simulink model "Paper_Simulation"  (R2020a)
settings: Solver=VariableStepAuto  StartTime=0.0  StopTime=1  RelTol=1e-3
model workspace (MAT data in the model file):
  Wo = 1
  wfinal = Simulink.Parameter
  wfinal.DataType = 'auto'
  wfinal.Dimensions = [0 0]
undefined symbols (not defined in the file): fdesignblkfcn, gcbh, T1, T2, Tf
libraries: powerlib_meascontrol x3, simulink x2, eeSinusoidalMeasurementV2 x1
settings Model: Creator=Ayush Agrawal  LastModifiedBy=Ayush Agrawal
settings DebuggingCC: AlgebraicLoopMsg=none

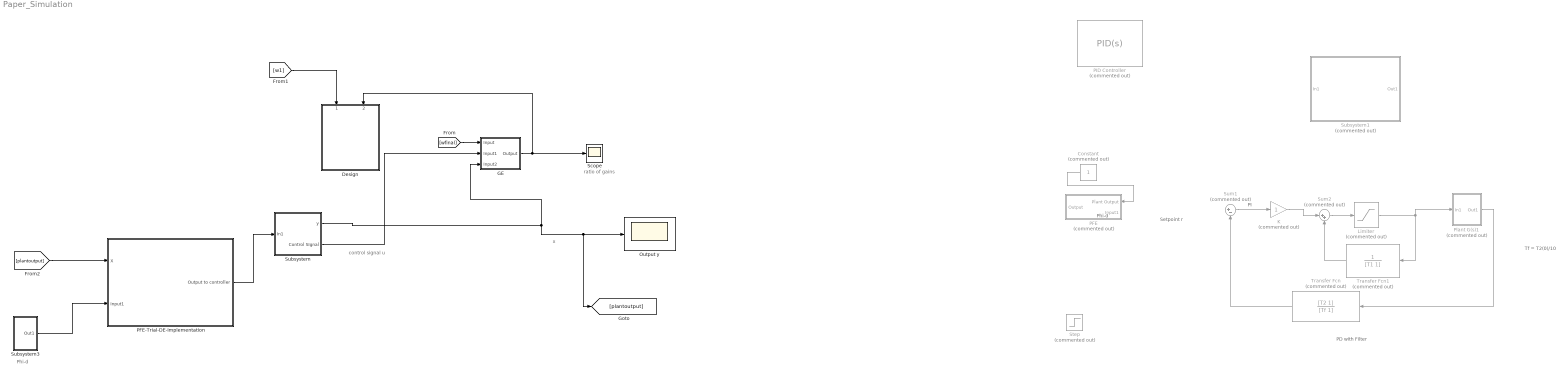
== system Paper_Simulation ==
  note: ratio of gains
  note: x
  note: Phi-d
  note: Phi-d
  note: control signal
      |         u
  note: Setpoint r
  note: PI
  note: PD with Filter
  note: Tf = T2(0)/10
  Constant : Constant  Commented=on
  Design : Subsystem  mask{a=1.5}
  GE : Subsystem  mask{winitial=10}
  K : Gain  Commented=on
  Limiter : Saturate  Commented=on
  Output y : Scope
  PFE : Subsystem  Commented=on
  PFE-Trial-DE-Implementation : Subsystem  mask{winitial=10}
  PID Controller : simulink/Continuous/PID Controller  Commented=on  Controller=PID  Form=Parallel  TimeDomain=Continuous-time  UseExternalTs=off  SampleTime=-1  IntegratorMethod=Forward Euler  FilterMethod=Forward Euler  ControllerParametersSource=internal  P=1  I=1  D=0  UseFilter=on  N=100  TunerSelectOption=Transfer Function Based (PID Tuner App)  InitialConditionSource=internal  InitialConditionForIntegrator=0  InitialConditionForFilter=0  DifferentiatorICPrevScaledInput=0  ExternalReset=none  TrackingMode=off  Kt=1  LimitOutput=off  UpperSaturationLimit=inf  LowerSaturationLimit=-inf  LinearizeAsGain=on  AntiWindupMode=none  Kb=1  POutMin=[]  POutMax=[]  IOutMin=[]  IOutMax=[]  DOutMin=[]  DOutMax=[]  NOutMin=[]  NOutMax=[]  SumOutMin=[]  SumOutMax=[]  SaturationOutMin=[]  SaturationOutMax=[]  PParamMin=[]  PParamMax=[]  IParamMin=[]  IParamMax=[]  DParamMin=[]  DParamMax=[]  NParamMin=[]  NParamMax=[]  KbParamMin=[]  KbParamMax=[]  KtParamMin=[]  KtParamMax=[]  KbOutMin=[]  KbOutMax=[]  KtOutMin=[]  KtOutMax=[]  IntegratorOutMin=[]  IntegratorOutMax=[]  FilterOutMin=[]  FilterOutMax=[]  SumI1OutMin=[]  SumI1OutMax=[]  SumI2OutMin=[]  SumI2OutMax=[]  SumI3OutMin=[]  SumI3OutMax=[]  SumI4OutMin=[]  SumI4OutMax=[]  SumDOutMin=[]  SumDOutMax=[]  DifferentiatorOutMin=[]  DifferentiatorOutMax=[]  FilterDiffOutCoefMin=[]  FilterDiffOutCoefMax=[]  ReciprocalOutMin=[]  ReciprocalOutMax=[]  SumDenOutMin=[]  SumDenOutMax=[]  SumNumOutMin=[]  SumNumOutMax=[]  DivideOutMin=[]  DivideOutMax=[]  UdiffTsProdOutMin=[]  UdiffTsProdOutMax=[]  NTsProdOutMin=[]  NTsProdOutMax=[]  UintegralTsProdOutMin=[]  UintegralTsProdOutMax=[]  UngainTsProdOutMin=[]  UngainTsProdOutMax=[]  IntegratorContinuousStateAttributes=''  IntegratorStateMustResolveToSignalObject=off  IntegratorRTWStateStorageClass=Auto  FilterContinuousStateAttributes=''  FilterStateMustResolveToSignalObject=off  FilterRTWStateStorageClass=Auto  ParallelPVariant=InternalParameters  IdealPVariant=Disabled  IVariant=InternalParameters  DVariant=InternalParameters  IntegratorVariant=Continuous  SatVariant=Disabled  AWVariant=Passthrough  PCopyVariant=Disabled  TRVariant=Disabled  FdbkBlocksVariant=Forward  IdealPFdbkVariant=Disabled  SatFdbkVariant=Disabled  DerivativeFilterVariant=ContFilter  NVariant=InternalParameters  NCopyVariant=Disabled  FilterICVariant=InternalICsFilter  IntegratorICVariant=InternalICs  ExternalResetVariant=Disabled  TRSumVariant=Passthrough  SumFdbkVariant=Disabled  SumVariant=Sum_PID  TsampFilterVariant=InternalTs  TsampNgainVariant=Passthrough  TsampIntegralVariant=Passthrough
  Plant G(s)1 : Subsystem  Commented=on
  Scope : Scope
  Step : Step  Commented=on  SampleTime=0
  Subsystem : Subsystem  mask{Ti=0, r=0.25}
  Subsystem1 : Subsystem  Commented=on
  Subsystem3 : Subsystem  mask{Phid=10}
      mask prompts: Phid "Phi-d"
  Sum1 : Sum  Commented=on  Inputs=|+-
  Sum2 : Sum  Commented=on  Inputs=|++
  Transfer Fcn : TransferFcn  Commented=on  Numerator=[T2 1]  Denominator=[Tf 1]
  Transfer Fcn1 : TransferFcn  Commented=on  Denominator=[T1 1]
  wires:
  Subsystem/1(y) -> GE/3(Input2), [plantoutput], Output y/1
  Sum2/1 -> Limiter/1
  Plant G(s)1/1(Out1) -> Transfer Fcn/1
  Limiter/1 -> Transfer Fcn1/1, Plant G(s)1/1(In1)
  Sum1/1 -> K/1
  Transfer Fcn/1 -> Sum1/2
  K/1 -> Sum2/1
  Transfer Fcn1/1 -> Sum2/2
  [wfinal] -> GE/1(Input)
  GE/1(Output) -> Scope/1, Design/2(Plant Gain Amplitude)
  [w1] -> Design/1(PFE O/P frequency)
  Constant/1 -> PFE/1(Plant Output)
  Subsystem3/1(Out1) -> PFE-Trial-DE-Implementation/2(Input1)
  [plantoutput] -> PFE-Trial-DE-Implementation/1(X)
  PFE-Trial-DE-Implementation/1(Output to controller) -> Subsystem/1(In1)
  Subsystem/2(Control SIgnal) -> GE/2(Input1)

== system Paper_Simulation/Design ==
  PFE O/P frequency : Inport
  Plant Gain Amplitude : Inport  Port=2
  Scope : Scope
  Scope1 : Scope
  Subsystem : Subsystem
  tag scope: K=global, Ti=global
  wires:
  PFE O/P frequency/1 -> Subsystem/1(PFE O/P freq)
  Plant Gain Amplitude/1 -> Subsystem/2(Input)
  Subsystem/1(K) -> Scope/1, [K]
  Subsystem/2(Ti) -> Scope1/1, [Ti]

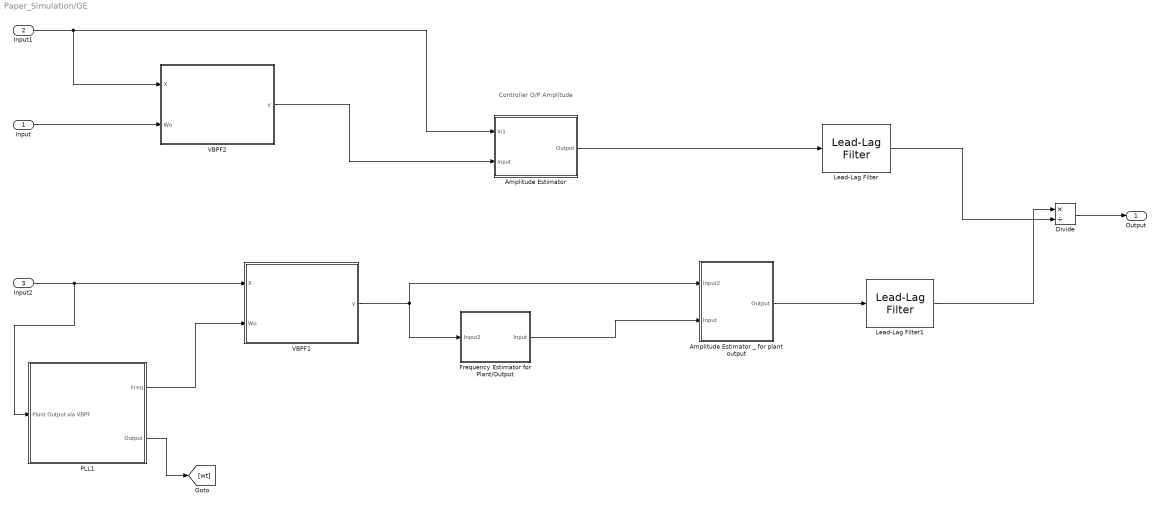
== system Paper_Simulation/GE ==
  note: Controller O/P Amplitude
  Input : Inport
  Input1 : Inport  Port=2
  Input2 : Inport  Port=3
  Amplitude Estimator : Subsystem
  Amplitude Estimator _ for plant output : Subsystem
  Divide : Product  Inputs=*/
  Frequency Estimator for Plant/Output : Subsystem
  Lead-Lag Filter : powerlib_meascontrol/Filters/Lead-Lag Filter  T1=0  T2=10/winitial  Vdc_Init=0  Ts=0
      settings: SourceProductBaseCode=PS
  Lead-Lag Filter1 : powerlib_meascontrol/Filters/Lead-Lag Filter  T1=0  T2=10/winitial  Vdc_Init=0  Ts=0
      settings: SourceProductBaseCode=PS
  PLL1 : Subsystem
  VBPF1 : Subsystem
  VBPF2 : Subsystem
  Output : Outport
  wires:
  Input1/1 -> VBPF2/1(X), Amplitude Estimator/1(In1)
  Input2/1 -> PLL1/1(Plant Output via VBPF), VBPF1/1(X)
  Amplitude Estimator/1(Output) -> Lead-Lag Filter/1
  Amplitude Estimator _ for plant output/1(Output) -> Lead-Lag Filter1/1
  Divide/1 -> Output/1
  Lead-Lag Filter1/1 -> Divide/1
  Lead-Lag Filter/1 -> Divide/2
  Frequency Estimator for Plant/Output/1(Input) -> Amplitude Estimator _ for plant output/2(Input)
  PLL1/1(Freq) -> VBPF1/2(Wo)
  PLL1/2(Output) -> [wt]
  Input/1 -> VBPF2/2(Wo)
  VBPF2/1(y) -> Amplitude Estimator/2(Input)
  VBPF1/1(y) -> Amplitude Estimator _ for plant output/1(Input2), Frequency Estimator for Plant/Output/1(Input2)

== system Paper_Simulation/PFE ==
  note: Phi-d
  Plant Output : Inport
  Input1 : Inport  Port=2
  PLL : Subsystem
  Subsystem : Subsystem  Commented=on
  Sum1 : Sum  Inputs=|+-
  VBPF1 : Subsystem
  Output : Outport
  wires:
  Plant Output/1 -> VBPF1/1(X)
  PLL/1(Output) -> Sum1/1
  Input1/1 -> Sum1/2
  Sum1/1 -> Output/1
  VBPF1/1(y) -> PLL/1(Plant Output via VBPF)

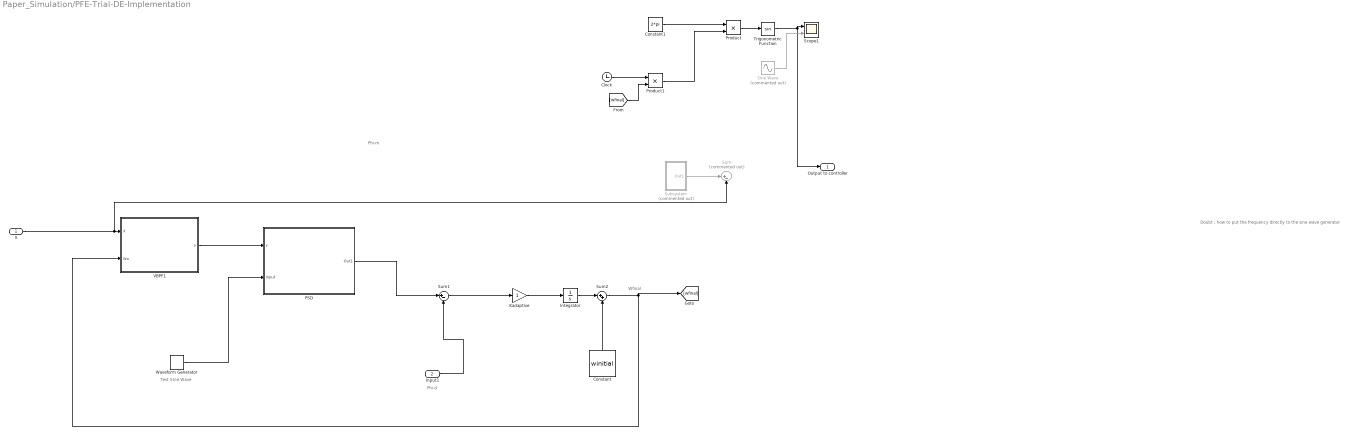
== system Paper_Simulation/PFE-Trial-DE-Implementation ==
  note: Phi-m
  note: Test SIne Wave
  note: Doubt : how to put the frequency directly to the sine wave generator
  note: Wfinal
  note: Phi-d
  X : Inport
  Input1 : Inport  Port=2
  Clock : Clock
  Constant : Constant  Value=winitial
  Constant1 : Constant  Value=2*pi
  Integrator : Integrator
  Kadaptive : Gain
  PSD : Subsystem
  Product : Product
  Product1 : Product
  Scope1 : Scope  NumInputPorts=2
  Sine Wave : Sin  Commented=on  Frequency=wfinal  SampleTime=0
  Subsystem : Subsystem  Commented=on  mask{wfinal=wfinal}
  Sum : Sum  Commented=on  Inputs=|+-
  Sum1 : Sum  Inputs=|+-
  Sum2 : Sum  Inputs=|++
  Trigonometric Function : Trigonometry
  VBPF1 : Subsystem
  Waveform Generator : simulink/Sources/Waveform Generator  OutMin=[]  OutMax=[]  OutDataTypeStr=double  SelectedSignal=1  Signals=sin(1,10,1)  BlockNames=MultiportSwitch_d946e39217074b0  SampleTime=0.1
  Output to controller : Outport
  wires:
  PSD/1(Out1) -> Sum1/1
  Input1/1 -> Sum1/2
  X/1 -> Sum/2, VBPF1/1(X)
  VBPF1/1(y) -> PSD/1(y)
  Waveform Generator/1 -> PSD/2(Input)
  Sum1/1 -> Kadaptive/1
  Kadaptive/1 -> Integrator/1
  Integrator/1 -> Sum2/1
  Constant/1 -> Sum2/2
  Sum2/1 -> VBPF1/2(Wo), [wfinal]
  Subsystem/1(Out1) -> Sum/1
  Product/1 -> Trigonometric Function/1
  Constant1/1 -> Product/1
  Clock/1 -> Product1/1
  Product1/1 -> Product/2
  Trigonometric Function/1 -> Output to controller/1, Scope1/1
  [wfinal] -> Product1/2
  Sine Wave/1 -> Scope1/2

== system Paper_Simulation/Plant G(s)1 ==
  In1 : Inport
  Out1 : Outport
  wires:
  In1/1 -> Out1/1

== system Paper_Simulation/Subsystem ==
  In1 : Inport
  Controller + Plant : Subsystem  mask{Td=Ti*r, Tf=Ti/20, T1=Ti/2, T2=Ti/2}
  y : Outport
  Control SIgnal : Outport  Port=2
  wires:
  Controller + Plant/1(y) -> y/1
  In1/1 -> Controller + Plant/1(In1)
  Controller + Plant/2(Control Signal) -> Control SIgnal/1

== system Paper_Simulation/Subsystem1 ==
  In1 : Inport
  Out1 : Outport
  wires:
  In1/1 -> Out1/1

== system Paper_Simulation/Subsystem3 ==
  Constant1 : Constant
  Out1 : Outport
  wires:
  Constant1/1 -> Out1/1

== system Paper_Simulation/Design/Subsystem ==
  note: Used for calculating P Gain for our controller
  note: Integral Time
  note: Plant Gain
  PFE O/P freq : Inport
  Input : Inport  Port=2
  Subsystem : Subsystem
  Subsystem1 : Subsystem
  K : Outport
  Ti : Outport  Port=2
  wires:
  Input/1 -> Subsystem/1(Plant Gain)
  Subsystem/1(K) -> K/1
  PFE O/P freq/1 -> Subsystem1/1(PFE O/P freq)
  Subsystem1/1(Ti) -> Ti/1

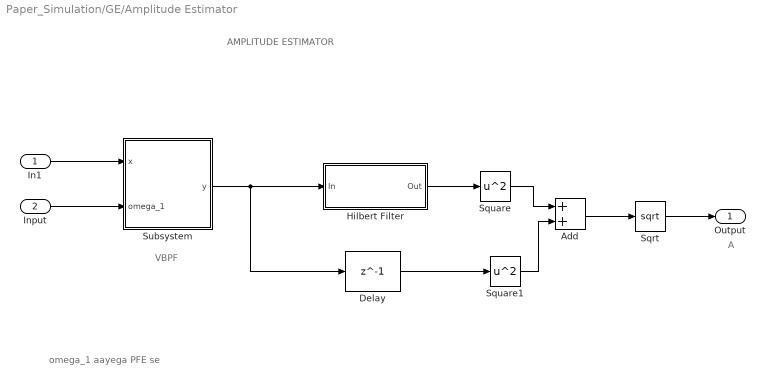
== system Paper_Simulation/GE/Amplitude Estimator ==
  note: omega_1 aayega PFE se
  note: A
  note: AMPLITUDE ESTIMATOR
  note: VBPF
  In1 : Inport
  Input : Inport  Port=2
  Add : Sum
  Delay : Delay  DelayLength=1  InitialCondition=0  UseCircularBuffer=on
  Hilbert Filter : Subsystem  DialogController=fdesignblkfcn  InitFcn=fdesignblkfcn(gcbh, {'InitFcn'});  mask(Hilbert Filter){}
      mask help: Design a Hilbert filter
      settings: CopyFcn=fdesignblkfcn(gcbh, {'CopyFcn'});
      mask Help: helpview(mapfilelocation('dsp'), 'dsphilbertfilter');
      mask Display: disp('Hilbert')
  Sqrt : Sqrt  SaturateOnIntegerOverflow=on
  Square : Math  Operator=square  SaturateOnIntegerOverflow=on
  Square1 : Math  Operator=square  SaturateOnIntegerOverflow=on
  Subsystem : Subsystem
  Output : Outport
  wires:
  Input/1 -> Subsystem/2(omega_1)
  In1/1 -> Subsystem/1(x)
  Subsystem/1(y) -> Delay/1, Hilbert Filter/1(In)
  Hilbert Filter/1(Out) -> Square/1
  Delay/1 -> Square1/1
  Square/1 -> Add/1
  Square1/1 -> Add/2
  Add/1 -> Sqrt/1
  Sqrt/1 -> Output/1

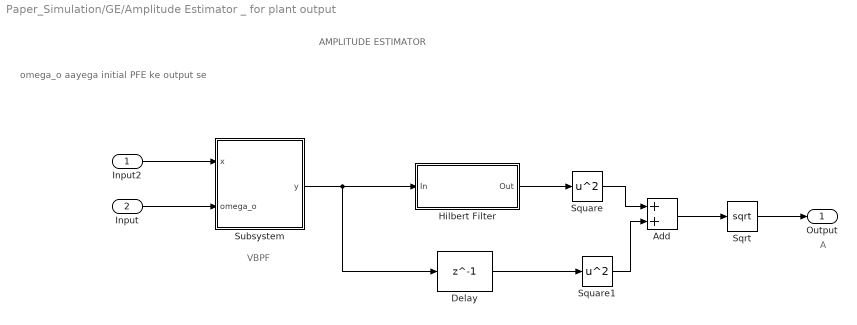
== system Paper_Simulation/GE/Amplitude Estimator _ for plant output ==
  note: omega_o aayega initial PFE ke output se
  note: A
  note: AMPLITUDE ESTIMATOR
  note: VBPF
  Input2 : Inport
  Input : Inport  Port=2
  Add : Sum
  Delay : Delay  DelayLength=1  InitialCondition=0  UseCircularBuffer=on
  Hilbert Filter : Subsystem  DialogController=fdesignblkfcn  InitFcn=fdesignblkfcn(gcbh, {'InitFcn'});  mask(Hilbert Filter){}
      mask help: Design a Hilbert filter
      settings: CopyFcn=fdesignblkfcn(gcbh, {'CopyFcn'});
      mask Help: helpview(mapfilelocation('dsp'), 'dsphilbertfilter');
      mask Display: disp('Hilbert')
  Sqrt : Sqrt  SaturateOnIntegerOverflow=on
  Square : Math  Operator=square  SaturateOnIntegerOverflow=on
  Square1 : Math  Operator=square  SaturateOnIntegerOverflow=on
  Subsystem : Subsystem
  Output : Outport
  wires:
  Input/1 -> Subsystem/2(omega_o)
  Input2/1 -> Subsystem/1(x)
  Subsystem/1(y) -> Delay/1, Hilbert Filter/1(In)
  Hilbert Filter/1(Out) -> Square/1
  Delay/1 -> Square1/1
  Square/1 -> Add/1
  Square1/1 -> Add/2
  Add/1 -> Sqrt/1
  Sqrt/1 -> Output/1

== system Paper_Simulation/GE/Frequency Estimator for Plant//Output ==
  Input2 : Inport
  PLL1 : Subsystem
  Input : Outport
  wires:
  Input2/1 -> PLL1/1(Plant Output via VBPF)
  PLL1/1(Freq) -> Input/1
  PLL1/2(Output) -> [wt]

== system Paper_Simulation/GE/PLL1 ==
  note: present phase
  Plant Output via VBPF : Inport
  Cos : Trigonometry  Operator=cos
  Integrator1 : Integrator
  PSD : Subsystem
  Transfer Fcn : TransferFcn  Numerator=[1 1]  Denominator=[1 1 0]
  Freq : Outport
  Output : Outport  Port=2
  wires:
  Cos/1 -> PSD/2(Input)
  PSD/1(Out1) -> Transfer Fcn/1
  Plant Output via VBPF/1 -> PSD/1(In1)
  Integrator1/1 -> Output/1, Cos/1
  Transfer Fcn/1 -> Freq/1, Integrator1/1

== system Paper_Simulation/GE/VBPF1 ==
  note: VBPF
  X : Inport
  Wo : Inport  Port=2
  Beta : Gain  Gain=0.15
  Integrator : Integrator
  Integrator1 : Integrator
  Product : Product
  Product1 : Product
  Sum : Sum  Inputs=|+-
  Sum1 : Sum  Inputs=|-+
  y : Outport
  wires:
  X/1 -> Sum/1
  Sum/1 -> Beta/1
  Integrator/1 -> Sum1/1
  Beta/1 -> Sum1/2
  Sum1/1 -> Product/1
  Wo/1 -> Product1/2, Product/2
  Product/1 -> Integrator1/1
  Integrator1/1 -> Product1/1, Sum/2, y/1
  Product1/1 -> Integrator/1

== system Paper_Simulation/GE/VBPF2 ==
  note: VBPF
  X : Inport
  Wo : Inport  Port=2
  Beta : Gain  Gain=1.5
  Integrator : Integrator
  Integrator1 : Integrator
  Product : Product
  Product1 : Product
  Sum : Sum  Inputs=|+-
  Sum1 : Sum  Inputs=|-+
  y : Outport
  wires:
  X/1 -> Sum/1
  Sum/1 -> Beta/1
  Integrator/1 -> Sum1/1
  Beta/1 -> Sum1/2
  Sum1/1 -> Product/1
  Wo/1 -> Product1/2, Product/2
  Product/1 -> Integrator1/1
  Integrator1/1 -> Product1/1, Sum/2, y/1
  Product1/1 -> Integrator/1

== system Paper_Simulation/PFE/PLL ==
  note: present phase
  Plant Output via VBPF : Inport
  Cos : Trigonometry  Operator=cos
  Integrator1 : Integrator
  PLL : powerlib_meascontrol/PLL/PLL  Fmin=45  Par_Init=[0, 60]  ParK=[180, 3200, 1]  TcD=1e-4  MaxRateChangeFreq=12  FilterCutOffFreq=25  Ts=0  AGC=on
      settings: SourceProductBaseCode=PS
  PSD : Subsystem
  Transfer Fcn : TransferFcn  Numerator=[1 1]  Denominator=[1 1 0]
  Output : Outport
  wires:
  Cos/1 -> PSD/2(Input)
  PSD/1(Out1) -> Transfer Fcn/1
  Plant Output via VBPF/1 -> PSD/1(In1)
  Integrator1/1 -> Output/1, Cos/1
  Transfer Fcn/1 -> Integrator1/1

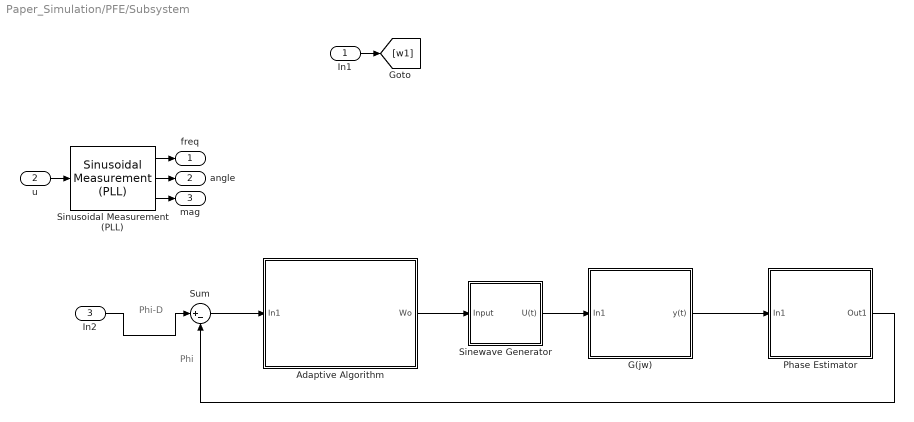
== system Paper_Simulation/PFE/Subsystem ==
  note: Phi
  note: Phi-D
  In1 : Inport
  u : Inport  Port=2
  In2 : Inport  Port=3
  Adaptive Algorithm : Subsystem
  G(jw) : Subsystem
  Phase Estimator : Subsystem
  Sinewave Generator : Subsystem
  Sinusoidal Measurement (PLL) : eeSinusoidalMeasurementV2/Sinusoidal Measurement (PLL)  Ki_PD=1000  Kp_LF=400  Ki_LF=20000  F0=60  Theta0=0  Mag0=1  Ts=-1
      settings: SourceProductBaseCode=PS
  Sum : Sum  Inputs=|+-
  freq : Outport
  angle : Outport  Port=2
  mag : Outport  Port=3
  wires:
  Phase Estimator/1(Out1) -> Sum/2
  Adaptive Algorithm/1(Wo) -> Sinewave Generator/1(Input)
  In2/1 -> Sum/1
  Sinusoidal Measurement (PLL)/2 -> angle/1
  Sinusoidal Measurement (PLL)/3 -> mag/1
  Sum/1 -> Adaptive Algorithm/1(In1)
  G(jw)/1(y(t)) -> Phase Estimator/1(In1)
  Sinusoidal Measurement (PLL)/1 -> freq/1
  Sinewave Generator/1(U(t)) -> G(jw)/1(In1)
  u/1 -> Sinusoidal Measurement (PLL)/1
  In1/1 -> [w1]

== system Paper_Simulation/PFE/VBPF1 ==
  note: VBPF
  X : Inport
  Wo : Inport  Port=2
  Beta : Gain
  Integrator : Integrator
  Integrator1 : Integrator
  Product : Product
  Product1 : Product
  Sum : Sum  Inputs=|+-
  Sum1 : Sum  Inputs=|-+
  y : Outport
  wires:
  X/1 -> Sum/1
  Sum/1 -> Beta/1
  Integrator/1 -> Sum1/1
  Beta/1 -> Sum1/2
  Sum1/1 -> Product/1
  Wo/1 -> Product1/2, Product/2
  Product/1 -> Integrator1/1
  Integrator1/1 -> Product1/1, Sum/2, y/1
  Product1/1 -> Integrator/1

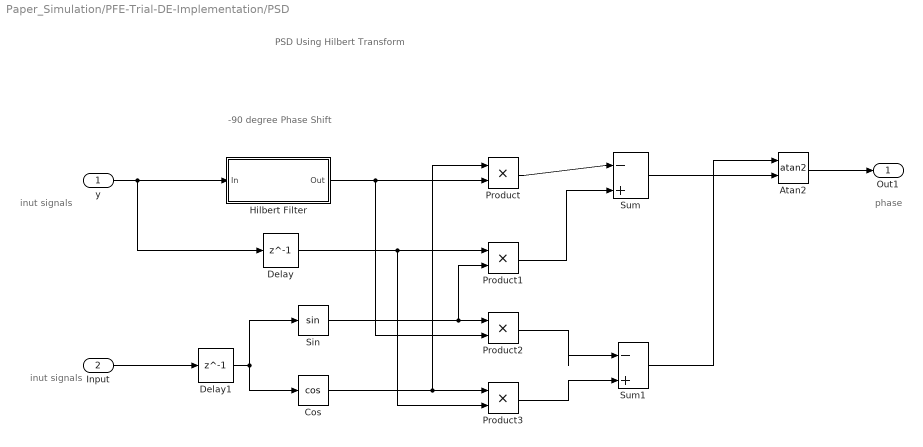
== system Paper_Simulation/PFE-Trial-DE-Implementation/PSD ==
  note: inut signals
  note: phase
  note: -90 degree Phase Shift
  note: PSD Using Hilbert Transform
  note: inut signals
  y : Inport
  Input : Inport  Port=2
  Atan2 : Trigonometry  Operator=atan2
  Cos : Trigonometry  Operator=cos
  Delay : Delay  DelayLength=1
  Delay1 : Delay  DelayLength=1
  Hilbert Filter : Subsystem  DialogController=fdesignblkfcn  InitFcn=fdesignblkfcn(gcbh, {'InitFcn'});  mask(Hilbert Filter){}
      mask help: Design a Hilbert filter
      settings: CopyFcn=fdesignblkfcn(gcbh, {'CopyFcn'});
      mask Help: helpview(mapfilelocation('dsp'), 'dsphilbertfilter');
      mask Display: disp('Hilbert')
  Product{,1..3} (4 alike) : Product
  Sin : Trigonometry
  Sum : Sum  Inputs=|-+
  Sum1 : Sum  Inputs=|-+
  Out1 : Outport
  wires:
  y/1 -> Delay/1, Hilbert Filter/1(In)
  Hilbert Filter/1(Out) -> Product2/2, Product/2
  Input/1 -> Delay1/1
  Delay1/1 -> Sin/1, Cos/1
  Sin/1 -> Product1/2, Product2/1
  Cos/1 -> Product/1, Product3/1
  Delay/1 -> Product3/2, Product1/1
  Product/1 -> Sum/1
  Product1/1 -> Sum/2
  Atan2/1 -> Out1/1
  Sum/1 -> Atan2/2
  Product2/1 -> Sum1/1
  Product3/1 -> Sum1/2
  Sum1/1 -> Atan2/1

== system Paper_Simulation/PFE-Trial-DE-Implementation/Subsystem ==
  Sine Wave : Sin  Frequency=wfinal  SampleTime=0
  Out1 : Outport
  wires:
  Sine Wave/1 -> Out1/1

== system Paper_Simulation/PFE-Trial-DE-Implementation/VBPF1 ==
  note: VBPF
  X : Inport
  Wo : Inport  Port=2
  Beta : Gain  Gain=1.5
  Integrator : Integrator
  Integrator1 : Integrator
  Product : Product
  Product1 : Product
  Sum : Sum  Inputs=|+-
  Sum1 : Sum  Inputs=|-+
  y : Outport
  wires:
  X/1 -> Sum/1
  Sum/1 -> Beta/1
  Integrator/1 -> Sum1/1
  Beta/1 -> Sum1/2
  Sum1/1 -> Product/1
  Wo/1 -> Product1/2, Product/2
  Product/1 -> Integrator1/1
  Integrator1/1 -> Product1/1, Sum/2, y/1
  Product1/1 -> Integrator/1

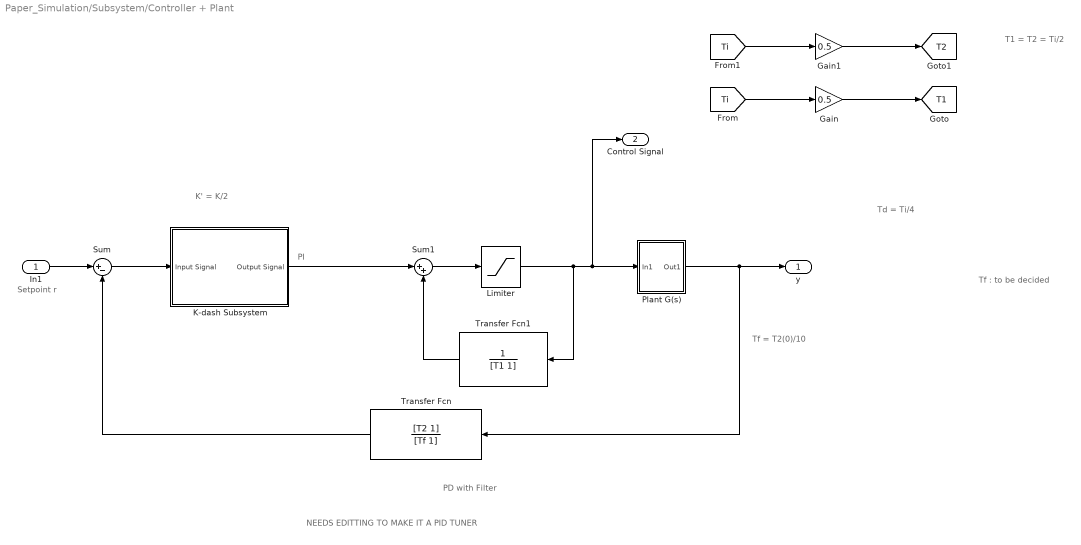
== system Paper_Simulation/Subsystem/Controller + Plant ==
  note: Tf : to be decided
  note: K' = K/2
  note: Td = Ti/4
  note: T1 = T2 = Ti/2
  note: NEEDS EDITTING TO MAKE IT A PID TUNER
  note: PI
  note: PD with Filter
  note: Setpoint r
  note: Tf = T2(0)/10
  In1 : Inport
  Gain : Gain  Gain=0.5
  Gain1 : Gain  Gain=0.5
  K-dash Subsystem : Subsystem
  Limiter : Saturate  UpperLimit=0.1  LowerLimit=-0.1  OutMin=-0.1  OutMax=0.1
  Plant G(s) : Subsystem
  Sum : Sum  Inputs=|+-
  Sum1 : Sum  Inputs=|++
  Transfer Fcn : TransferFcn  Numerator=[T2 1]  Denominator=[Tf 1]
  Transfer Fcn1 : TransferFcn  Denominator=[T1 1]
  y : Outport
  Control Signal : Outport  Port=2
  tag scope: T1=global, T2=global
  wires:
  Sum/1 -> K-dash Subsystem/1(Input Signal)
  Sum1/1 -> Limiter/1
  Limiter/1 -> Transfer Fcn1/1, Control Signal/1, Plant G(s)/1(In1)
  Transfer Fcn1/1 -> Sum1/2
  In1/1 -> Sum/1
  K-dash Subsystem/1(Output Signal) -> Sum1/1
  Plant G(s)/1(Out1) -> Transfer Fcn/1, y/1
  Transfer Fcn/1 -> Sum/2
  [Ti] -> Gain/1
  Gain/1 -> [T1]
  Gain1/1 -> [T2]
  [Ti] -> Gain1/1

== system Paper_Simulation/Design/Subsystem/Subsystem ==
  Plant Gain : Inport
  Constant : Constant  Value=a
  Constant1 : Constant
  Divide : Product  Inputs=/
  Product : Product
  Sqrt : Sqrt  SaturateOnIntegerOverflow=on
  Square : Math  Operator=square  SaturateOnIntegerOverflow=on
  Sum : Sum  Inputs=|++
  K : Outport
  wires:
  Divide/1 -> K/1
  Sum/1 -> Sqrt/1
  Square/1 -> Sum/1
  Sqrt/1 -> Product/1
  Plant Gain/1 -> Product/2
  Constant/1 -> Square/1
  Product/1 -> Divide/1
  Constant1/1 -> Sum/2

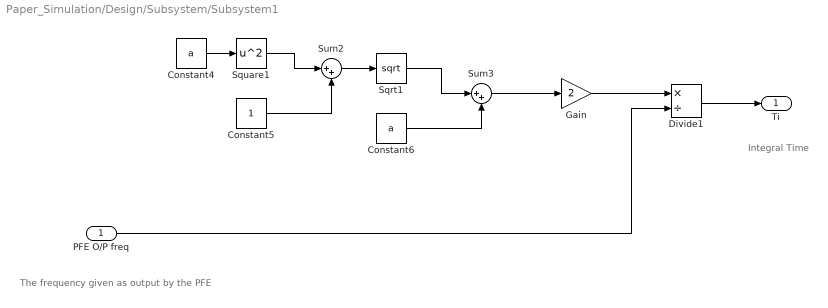
== system Paper_Simulation/Design/Subsystem/Subsystem1 ==
  note: Integral Time
  note: The frequency given as output by the PFE
  PFE O/P freq : Inport
  Constant4 : Constant  Value=a
  Constant5 : Constant
  Constant6 : Constant  Value=a
  Divide1 : Product  Inputs=*/
  Gain : Gain  Gain=2
  Sqrt1 : Sqrt  SaturateOnIntegerOverflow=on
  Square1 : Math  Operator=square  SaturateOnIntegerOverflow=on
  Sum2 : Sum  Inputs=|++
  Sum3 : Sum  Inputs=|++
  Ti : Outport
  wires:
  Constant6/1 -> Sum3/2
  PFE O/P freq/1 -> Divide1/2
  Sum3/1 -> Gain/1
  Gain/1 -> Divide1/1
  Sum2/1 -> Sqrt1/1
  Constant5/1 -> Sum2/2
  Constant4/1 -> Square1/1
  Sqrt1/1 -> Sum3/1
  Square1/1 -> Sum2/1
  Divide1/1 -> Ti/1

== system Paper_Simulation/GE/Amplitude Estimator/Hilbert Filter ==
  In : Inport
  Generated Filter Block : DiscreteFir  Tag=BlockMethodSubSystem  Coefficients=[-0.026449858259791379 -0.00578355491829027 -0.016572261903348456 -0.0095390561131982743 -0.022461390535071568 -0.014999256435125952 -0.030323967074738556 -0.023012528163449009 -0.041429315821655127 -0.035762828939278346 -0.05911752381753177 -0.059034685410808696 -0.094459906652176406 -0.11739830204172252 -0.21797718993610349 -0.62869353747279177 0.62869353747279177 0.21797718993610349 0.11739830204172252 0.094459906652176406 0.059034685410808696 0.05911752381753177 0.035762828939278346 0.041429315821655127 0.023012528163449009 0.030323967074738556 0.014999256435125952 0.022461390535071568 0.0095390561131982743 0.016572261903348456 0.00578355491829027 0.026449858259791379]  InputProcessing=Columns as channels (frame based)
  Out : Outport  VectorParamsAs1DForOutWhenUnconnected=off
  wires:
  Generated Filter Block/1 -> Out/1
  In/1 -> Generated Filter Block/1

== system Paper_Simulation/GE/Amplitude Estimator/Subsystem ==
  x : Inport
  omega_1 : Inport  Port=2
  VBPF : Subsystem
  y : Outport
  wires:
  omega_1/1 -> VBPF/2(W1)
  x/1 -> VBPF/1(X)
  VBPF/1(y) -> y/1

== system Paper_Simulation/GE/Amplitude Estimator _ for plant output/Hilbert Filter ==
  In : Inport
  Generated Filter Block : DiscreteFir  Tag=BlockMethodSubSystem  Coefficients=[-0.026449858259791379 -0.00578355491829027 -0.016572261903348456 -0.0095390561131982743 -0.022461390535071568 -0.014999256435125952 -0.030323967074738556 -0.023012528163449009 -0.041429315821655127 -0.035762828939278346 -0.05911752381753177 -0.059034685410808696 -0.094459906652176406 -0.11739830204172252 -0.21797718993610349 -0.62869353747279177 0.62869353747279177 0.21797718993610349 0.11739830204172252 0.094459906652176406 0.059034685410808696 0.05911752381753177 0.035762828939278346 0.041429315821655127 0.023012528163449009 0.030323967074738556 0.014999256435125952 0.022461390535071568 0.0095390561131982743 0.016572261903348456 0.00578355491829027 0.026449858259791379]  InputProcessing=Columns as channels (frame based)
  Out : Outport  VectorParamsAs1DForOutWhenUnconnected=off
  wires:
  Generated Filter Block/1 -> Out/1
  In/1 -> Generated Filter Block/1

== system Paper_Simulation/GE/Amplitude Estimator _ for plant output/Subsystem ==
  x : Inport
  omega_o : Inport  Port=2
  VBPF : Subsystem
  y : Outport
  wires:
  omega_o/1 -> VBPF/2(wo)
  x/1 -> VBPF/1(X)
  VBPF/1(y) -> y/1

== system Paper_Simulation/GE/Frequency Estimator for Plant//Output/PLL1 ==
  note: present phase
  Plant Output via VBPF : Inport
  Cos : Trigonometry  Operator=cos
  Integrator1 : Integrator
  PSD : Subsystem
  Transfer Fcn : TransferFcn  Numerator=[1 1]  Denominator=[1 1 0]
  Freq : Outport
  Output : Outport  Port=2
  wires:
  Cos/1 -> PSD/2(Input)
  PSD/1(Out1) -> Transfer Fcn/1
  Plant Output via VBPF/1 -> PSD/1(In1)
  Integrator1/1 -> Output/1, Cos/1
  Transfer Fcn/1 -> Freq/1, Integrator1/1

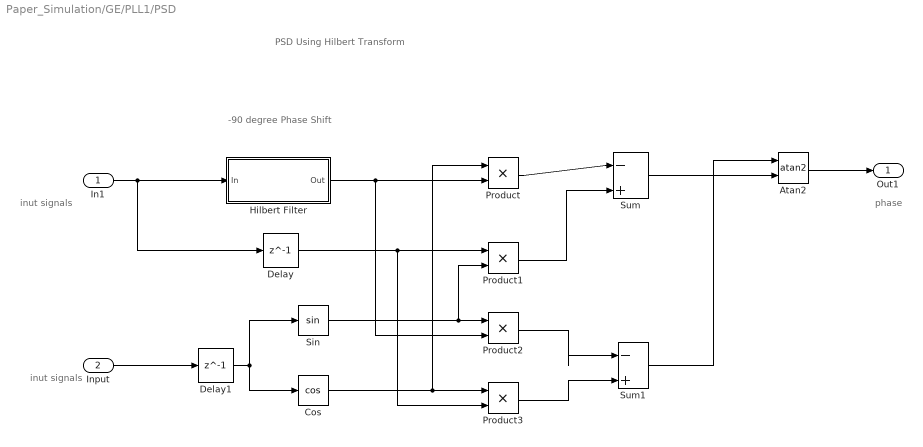
== system Paper_Simulation/GE/PLL1/PSD ==
  note: inut signals
  note: phase
  note: -90 degree Phase Shift
  note: PSD Using Hilbert Transform
  note: inut signals
  In1 : Inport
  Input : Inport  Port=2
  Atan2 : Trigonometry  Operator=atan2
  Cos : Trigonometry  Operator=cos
  Delay : Delay  DelayLength=1
  Delay1 : Delay  DelayLength=1
  Hilbert Filter : Subsystem  DialogController=fdesignblkfcn  InitFcn=fdesignblkfcn(gcbh, {'InitFcn'});  mask(Hilbert Filter){}
      mask help: Design a Hilbert filter
      settings: CopyFcn=fdesignblkfcn(gcbh, {'CopyFcn'});
      mask Help: helpview(mapfilelocation('dsp'), 'dsphilbertfilter');
      mask Display: disp('Hilbert')
  Product{,1..3} (4 alike) : Product
  Sin : Trigonometry
  Sum : Sum  Inputs=|-+
  Sum1 : Sum  Inputs=|-+
  Out1 : Outport
  wires:
  In1/1 -> Delay/1, Hilbert Filter/1(In)
  Hilbert Filter/1(Out) -> Product2/2, Product/2
  Input/1 -> Delay1/1
  Delay1/1 -> Sin/1, Cos/1
  Sin/1 -> Product1/2, Product2/1
  Cos/1 -> Product/1, Product3/1
  Delay/1 -> Product3/2, Product1/1
  Product/1 -> Sum/1
  Product1/1 -> Sum/2
  Atan2/1 -> Out1/1
  Sum/1 -> Atan2/2
  Product2/1 -> Sum1/1
  Product3/1 -> Sum1/2
  Sum1/1 -> Atan2/1

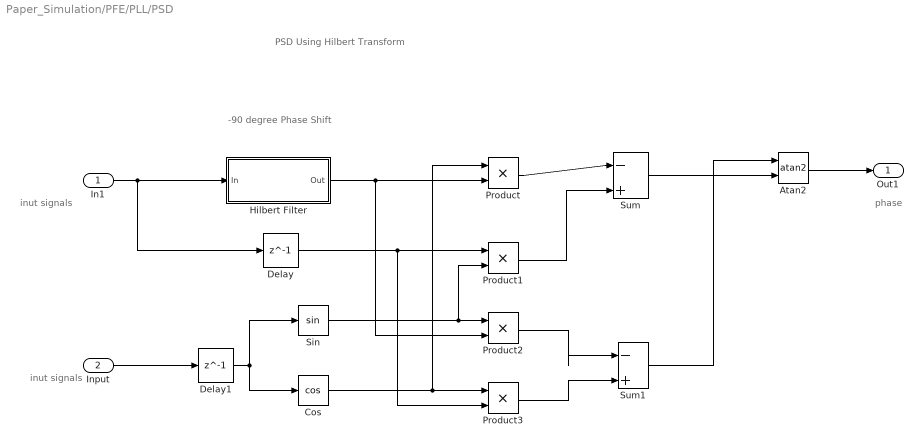
== system Paper_Simulation/PFE/PLL/PSD ==
  note: inut signals
  note: phase
  note: -90 degree Phase Shift
  note: PSD Using Hilbert Transform
  note: inut signals
  In1 : Inport
  Input : Inport  Port=2
  Atan2 : Trigonometry  Operator=atan2
  Cos : Trigonometry  Operator=cos
  Delay : Delay  DelayLength=1
  Delay1 : Delay  DelayLength=1
  Hilbert Filter : Subsystem  DialogController=fdesignblkfcn  InitFcn=fdesignblkfcn(gcbh, {'InitFcn'});  mask(Hilbert Filter){}
      mask help: Design a Hilbert filter
      settings: CopyFcn=fdesignblkfcn(gcbh, {'CopyFcn'});
      mask Help: helpview(mapfilelocation('dsp'), 'dsphilbertfilter');
      mask Display: disp('Hilbert')
  Product{,1..3} (4 alike) : Product
  Sin : Trigonometry
  Sum : Sum  Inputs=|-+
  Sum1 : Sum  Inputs=|-+
  Out1 : Outport
  wires:
  In1/1 -> Delay/1, Hilbert Filter/1(In)
  Hilbert Filter/1(Out) -> Product2/2, Product/2
  Input/1 -> Delay1/1
  Delay1/1 -> Sin/1, Cos/1
  Sin/1 -> Product1/2, Product2/1
  Cos/1 -> Product/1, Product3/1
  Delay/1 -> Product3/2, Product1/1
  Product/1 -> Sum/1
  Product1/1 -> Sum/2
  Atan2/1 -> Out1/1
  Sum/1 -> Atan2/2
  Product2/1 -> Sum1/1
  Product3/1 -> Sum1/2
  Sum1/1 -> Atan2/1

== system Paper_Simulation/PFE/Subsystem/Adaptive Algorithm ==
  In1 : Inport
  Wo : Outport
  wires:
  In1/1 -> Wo/1

== system Paper_Simulation/PFE/Subsystem/G(jw) ==
  In1 : Inport
  y(t) : Outport

== system Paper_Simulation/PFE/Subsystem/Phase Estimator ==
  In1 : Inport
  Out1 : Outport
  wires:
  In1/1 -> Out1/1

== system Paper_Simulation/PFE/Subsystem/Sinewave Generator ==
  Input : Inport
  U(t) : Outport

== system Paper_Simulation/PFE-Trial-DE-Implementation/PSD/Hilbert Filter ==
  In : Inport
  Generated Filter Block : DiscreteFir  Tag=BlockMethodSubSystem  Coefficients=[5.22597433146325396e-16 -0.0960625074558433545 -6.53552528176760002e-16 -0.073873596707413447 -1.60565794691115825e-18 -0.114550630898285405 -2.2487890416571374e-16 -0.204297562619966455 7.44886168555606983e-17 -0.633937925126545787 0 0.633937925126545787 -7.44886168555606983e-17 0.204297562619966455 2.2487890416571374e-16 0.114550630898285405 1.60565794691115825e-18 0.073873596707413447 6.53552528176760002e-16 0.0960625074558433545 -5.22597433146325396e-16]  InputProcessing=Columns as channels (frame based)
  Out : Outport  VectorParamsAs1DForOutWhenUnconnected=off
  wires:
  Generated Filter Block/1 -> Out/1
  In/1 -> Generated Filter Block/1

== system Paper_Simulation/Subsystem/Controller + Plant/K-dash Subsystem ==
  Input Signal : Inport
  Gain : Gain  Gain=0.5
  Product : Product
  Output Signal : Outport
  tag scope: Kdash=global
  wires:
  Gain/1 -> Product/1, [Kdash]
  [K] -> Gain/1
  Input Signal/1 -> Product/2
  Product/1 -> Output Signal/1

== system Paper_Simulation/Subsystem/Controller + Plant/Plant G(s) ==
  In1 : Inport
  Plant G(s) : Subsystem
  Out1 : Outport
  wires:
  In1/1 -> Plant G(s)/1(Input1)
  Plant G(s)/1(Input2) -> Out1/1

== system Paper_Simulation/GE/Amplitude Estimator/Subsystem/VBPF ==
  note: W1 from PFE
  note: USES OF VBPF
  note: (i) elimination of DC Values
      | (ii) attenuation of harmonics, arising for example if there
      | are nonlinearities in the plant or actuator
      | (iii) reduction in the effect of additive noise.
  note: VBPF
  X : Inport
  W1 : Inport  Port=2
  Beta : Gain  Gain=0.15
  Integrator : Integrator
  Integrator1 : Integrator
  Product : Product
  Product1 : Product
  Sum : Sum  Inputs=|+-
  Sum1 : Sum  Inputs=|-+
  y : Outport
  wires:
  X/1 -> Sum/1
  Sum/1 -> Beta/1
  Integrator/1 -> Sum1/1
  Beta/1 -> Sum1/2
  Sum1/1 -> Product/1
  W1/1 -> Product1/2, Product/2
  Product/1 -> Integrator1/1
  Integrator1/1 -> Product1/1, Sum/2, y/1
  Product1/1 -> Integrator/1

== system Paper_Simulation/GE/Amplitude Estimator _ for plant output/Subsystem/VBPF ==
  note: USES OF VBPF
  note: (i) elimination of DC Values
      | (ii) attenuation of harmonics, arising for example if there
      | are nonlinearities in the plant or actuator
      | (iii) reduction in the effect of additive noise.
  note: VBPF
  X : Inport
  wo : Inport  Port=2
  Beta : Gain  Gain=0.15
  Integrator : Integrator
  Integrator1 : Integrator
  Product : Product
  Product1 : Product
  Sum : Sum  Inputs=|+-
  Sum1 : Sum  Inputs=|-+
  y : Outport
  wires:
  X/1 -> Sum/1
  Sum/1 -> Beta/1
  Integrator/1 -> Sum1/1
  Beta/1 -> Sum1/2
  Sum1/1 -> Product/1
  wo/1 -> Product1/2, Product/2
  Product/1 -> Integrator1/1
  Integrator1/1 -> Product1/1, Sum/2, y/1
  Product1/1 -> Integrator/1

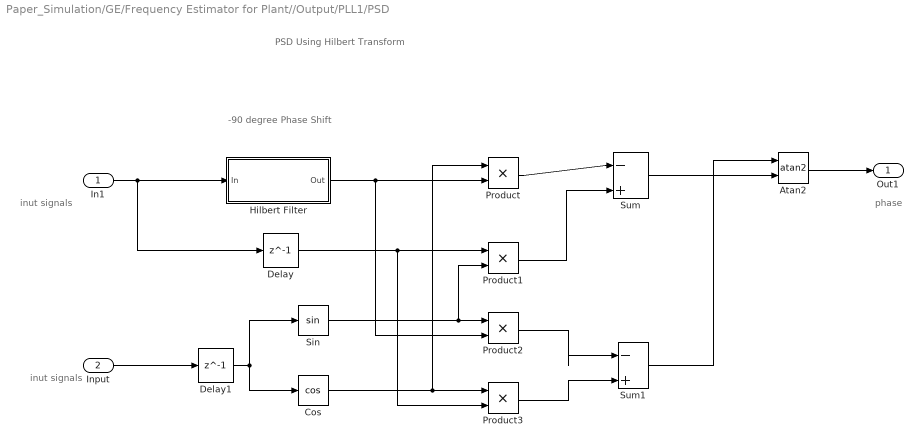
== system Paper_Simulation/GE/Frequency Estimator for Plant//Output/PLL1/PSD ==
  note: inut signals
  note: phase
  note: -90 degree Phase Shift
  note: PSD Using Hilbert Transform
  note: inut signals
  In1 : Inport
  Input : Inport  Port=2
  Atan2 : Trigonometry  Operator=atan2
  Cos : Trigonometry  Operator=cos
  Delay : Delay  DelayLength=1
  Delay1 : Delay  DelayLength=1
  Hilbert Filter : Subsystem  DialogController=fdesignblkfcn  InitFcn=fdesignblkfcn(gcbh, {'InitFcn'});  mask(Hilbert Filter){}
      mask help: Design a Hilbert filter
      settings: CopyFcn=fdesignblkfcn(gcbh, {'CopyFcn'});
      mask Help: helpview(mapfilelocation('dsp'), 'dsphilbertfilter');
      mask Display: disp('Hilbert')
  Product{,1..3} (4 alike) : Product
  Sin : Trigonometry
  Sum : Sum  Inputs=|-+
  Sum1 : Sum  Inputs=|-+
  Out1 : Outport
  wires:
  In1/1 -> Delay/1, Hilbert Filter/1(In)
  Hilbert Filter/1(Out) -> Product2/2, Product/2
  Input/1 -> Delay1/1
  Delay1/1 -> Sin/1, Cos/1
  Sin/1 -> Product1/2, Product2/1
  Cos/1 -> Product/1, Product3/1
  Delay/1 -> Product3/2, Product1/1
  Product/1 -> Sum/1
  Product1/1 -> Sum/2
  Atan2/1 -> Out1/1
  Sum/1 -> Atan2/2
  Product2/1 -> Sum1/1
  Product3/1 -> Sum1/2
  Sum1/1 -> Atan2/1

== system Paper_Simulation/GE/PLL1/PSD/Hilbert Filter ==
  In : Inport
  Generated Filter Block : DiscreteFir  Tag=BlockMethodSubSystem  Coefficients=[-0.026449858259791379 -0.00578355491829027 -0.016572261903348456 -0.0095390561131982743 -0.022461390535071568 -0.014999256435125952 -0.030323967074738556 -0.023012528163449009 -0.041429315821655127 -0.035762828939278346 -0.05911752381753177 -0.059034685410808696 -0.094459906652176406 -0.11739830204172252 -0.21797718993610349 -0.62869353747279177 0.62869353747279177 0.21797718993610349 0.11739830204172252 0.094459906652176406 0.059034685410808696 0.05911752381753177 0.035762828939278346 0.041429315821655127 0.023012528163449009 0.030323967074738556 0.014999256435125952 0.022461390535071568 0.0095390561131982743 0.016572261903348456 0.00578355491829027 0.026449858259791379]  InputProcessing=Columns as channels (frame based)
  Out : Outport  VectorParamsAs1DForOutWhenUnconnected=off
  wires:
  Generated Filter Block/1 -> Out/1
  In/1 -> Generated Filter Block/1

== system Paper_Simulation/PFE/PLL/PSD/Hilbert Filter ==
  In : Inport
  Generated Filter Block : DiscreteFir  Tag=BlockMethodSubSystem  Coefficients=[-0.026449858259791379 -0.00578355491829027 -0.016572261903348456 -0.0095390561131982743 -0.022461390535071568 -0.014999256435125952 -0.030323967074738556 -0.023012528163449009 -0.041429315821655127 -0.035762828939278346 -0.05911752381753177 -0.059034685410808696 -0.094459906652176406 -0.11739830204172252 -0.21797718993610349 -0.62869353747279177 0.62869353747279177 0.21797718993610349 0.11739830204172252 0.094459906652176406 0.059034685410808696 0.05911752381753177 0.035762828939278346 0.041429315821655127 0.023012528163449009 0.030323967074738556 0.014999256435125952 0.022461390535071568 0.0095390561131982743 0.016572261903348456 0.00578355491829027 0.026449858259791379]  InputProcessing=Columns as channels (frame based)
  Out : Outport  VectorParamsAs1DForOutWhenUnconnected=off
  wires:
  Generated Filter Block/1 -> Out/1
  In/1 -> Generated Filter Block/1

== system Paper_Simulation/Subsystem/Controller + Plant/Plant G(s)/Plant G(s) ==
  Input1 : Inport
  Transfer Fcn : TransferFcn  Denominator=[1 1.5 1]
  Input2 : Outport
  wires:
  Input1/1 -> Transfer Fcn/1
  Transfer Fcn/1 -> Input2/1

== system Paper_Simulation/GE/Frequency Estimator for Plant//Output/PLL1/PSD/Hilbert Filter ==
  In : Inport
  Generated Filter Block : DiscreteFir  Tag=BlockMethodSubSystem  Coefficients=[-0.026449858259791379 -0.00578355491829027 -0.016572261903348456 -0.0095390561131982743 -0.022461390535071568 -0.014999256435125952 -0.030323967074738556 -0.023012528163449009 -0.041429315821655127 -0.035762828939278346 -0.05911752381753177 -0.059034685410808696 -0.094459906652176406 -0.11739830204172252 -0.21797718993610349 -0.62869353747279177 0.62869353747279177 0.21797718993610349 0.11739830204172252 0.094459906652176406 0.059034685410808696 0.05911752381753177 0.035762828939278346 0.041429315821655127 0.023012528163449009 0.030323967074738556 0.014999256435125952 0.022461390535071568 0.0095390561131982743 0.016572261903348456 0.00578355491829027 0.026449858259791379]  InputProcessing=Columns as channels (frame based)
  Out : Outport  VectorParamsAs1DForOutWhenUnconnected=off
  wires:
  Generated Filter Block/1 -> Out/1
  In/1 -> Generated Filter Block/1
